simulink model "differential_solver"  (R2021a)
settings: Solver=VariableStepAuto  StartTime=0.0  StopTime=10.0  RelTol=1e-3
settings Model: Creator=Davie  LastModifiedBy=Davie

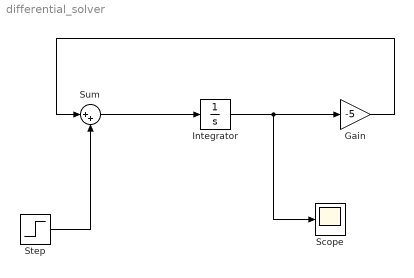
== system differential_solver ==
  Gain : Gain  Gain=-5
  Integrator : Integrator  InitialCondition=-2
  Scope : Scope
  Step : Step  SampleTime=0
  Sum : Sum  Inputs=|++
  wires:
  Step/1 -> Sum/2
  Gain/1 -> Sum/1
  Integrator/1 -> Scope/1, Gain/1
  Sum/1 -> Integrator/1
